simulink model "ex1"  (Simulink 7.9)
settings: Solver=ode45  StartTime=0.0  StopTime=10.0  RelTol=1e-3
settings Model: Creator=Cristi  LastModifiedBy=Cristi

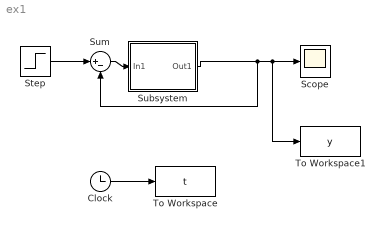
== system ex1 ==
  Clock : Clock
  Scope : Scope
  Step : Step  SampleTime=0
  Subsystem : Subsystem  mask{a=12}
      mask prompts: a "val lui a"
      mask CallbackString:
      | if str2num(get_param(gcb,'a'))<0
      |     error('negativa!!!')
      | end
  Sum : Sum  Inputs=|+-
  To Workspace : ToWorkspace  VariableName=t  SampleTime=-1
  To Workspace1 : ToWorkspace  VariableName=y  SampleTime=-1
  wires:
  Step/1 -> Sum/1
  Subsystem/1(Out1) -> To Workspace1/1, Scope/1, Sum/2
  Sum/1 -> Subsystem/1(In1)
  Clock/1 -> To Workspace/1

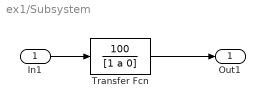
== system ex1/Subsystem ==
  In1 : Inport
  Transfer Fcn : TransferFcn  Numerator=[100]  Denominator=[1 a 0]
  Out1 : Outport
  wires:
  Transfer Fcn/1 -> Out1/1
  In1/1 -> Transfer Fcn/1
